simulink model "test_angular_velocity"  (Simulink 8.3)
settings: Solver=ode45  StartTime=0.0  StopTime=2  MaxStep=Step_Time  RelTol=1e-3
settings Model: Creator=saeed  LastModifiedBy=milad
settings OptimizationCC: ExpressionDepthLimit=2147483647
settings DebuggingCC: FcnCallInpInsideContextMsg=UseLocalSettings  FrameProcessingCompatibilityMsg=error
settings ConfigComp: CovMetricSettings=dw  CovHtmlReporting=on  CovSaveCumulativeToWorkspaceVar=on  CovSaveSingleToWorkspaceVar=on  CovModelRefEnable=Off  CovExternalEMLEnable=off

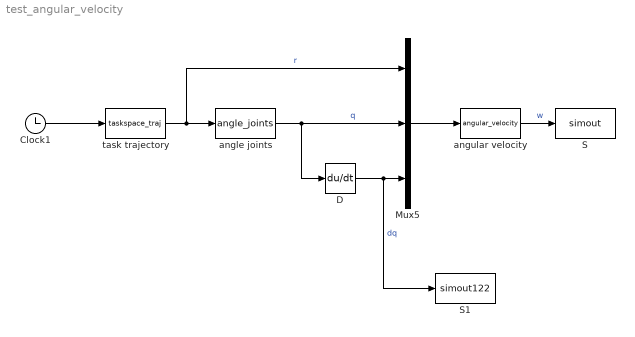
== system test_angular_velocity ==
  Clock1 : Clock
  D : Derivative
  Mux5 : Mux  Inputs=3
  S : ToWorkspace  VariableName=simout  SaveFormat=Structure With Time  SampleTime=-1
  S1 : ToWorkspace  VariableName=simout122  SaveFormat=Structure With Time  SampleTime=-1
  angle joints : MATLABFcn  MATLABFcn=angle_joints
  angular velocity : MATLABFcn  MATLABFcn=angular_velocity
  task trajectory : MATLABFcn  MATLABFcn=taskspace_traj
  wires:
  angular velocity/1 -> S/1  "w"
  Clock1/1 -> task trajectory/1
  task trajectory/1 -> Mux5/1, angle joints/1  "r"
  angle joints/1 -> Mux5/2, D/1  "q"
  D/1 -> S1/1, Mux5/3  "dq"
  Mux5/1 -> angular velocity/1
